simulink model "stage_2"  (Simulink 8.7)
settings: Solver=VariableStepAuto  StartTime=0.0  StopTime=inf  FixedStep=.000295  MaxStep=.0000118  RelTol=1e-3
settings Model: Creator=eispin  LastModifiedBy=eispin  PauseTimes=0
settings DataIOCC: LimitDataPoints=off  SaveFormat=Dataset
settings DebuggingCC: UnderspecifiedInitializationDetection=Simplified  MergeDetectMultiDrivingBlocksExec=error
settings HardwareCC: ProdBitPerPointer=64  ProdLargestAtomicFloat=Float  ProdIntDivRoundTo=Zero  ProdEndianess=LittleEndian  ProdWordSize=64  ProdHWDeviceType=Intel->x86-64 (Windows64)
settings ModelReferenceCC: PropagateSignalLabelsOutOfModel=on
settings ConfigComp: CovModelRefEnable=off

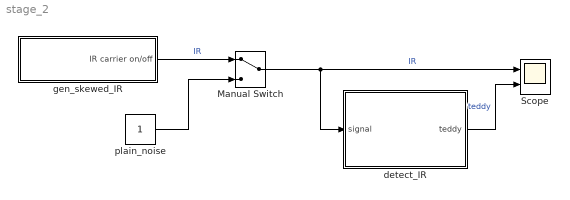
== system stage_2 ==
  Manual Switch : ManualSwitch
  Scope : Scope  NumInputPorts=2
  detect_IR : Stateflow chart  TreatAsAtomicUnit=on
  gen_skewed_IR : Subsystem
  plain_noise : Constant
  wires:
  Manual Switch/1 -> detect_IR/1(signal), Scope/1  "IR"
  detect_IR/1(teddy) -> Scope/2  "teddy"
  gen_skewed_IR/1(IR carrier on/off) -> Manual Switch/1  "IR"
  plain_noise/1 -> Manual Switch/2

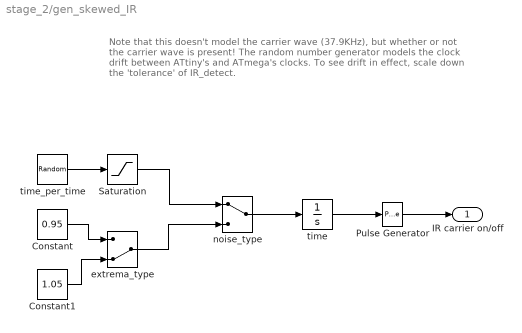
== system stage_2/gen_skewed_IR ==
  note: Note that this doesn't model the carrier wave (37.9KHz),
      | but whether or not the carrier wave is present!
      | The random number generator models the clock drift
      | between ATtiny's and ATmega's clocks.
      | To see drift in effect, scale down the 'tolerance' of IR_detect.
  Constant : Constant  Value=0.95
  Constant1 : Constant  Value=1.05
  Pulse Generator : DiscretePulseGenerator  PulseType=Time based  TimeSource=Use external signal  Period=.001180  PulseWidth=50
  Saturation : Saturate  UpperLimit=1.05  LowerLimit=0.95
  extrema_type : ManualSwitch  CurrentSetting=0
  noise_type : ManualSwitch
  time : Integrator
  time_per_time : RandomNumber  Mean=1  Variance=0.05  Seed=1337  SampleTime=0.000059
  IR carrier on/off : Outport
  wires:
  Pulse Generator/1 -> IR carrier on/off/1
  time/1 -> Pulse Generator/1
  time_per_time/1 -> Saturation/1
  noise_type/1 -> time/1
  Saturation/1 -> noise_type/1
  Constant/1 -> extrema_type/1
  extrema_type/1 -> noise_type/2
  Constant1/1 -> extrema_type/2

== stateflow chart detect_IR ==
  state NoTeddy
    % signal is 1,
    % waiting for 0
    entry:
    teddy = 0
  state Something
    % signal is 0,
    % waiting for 1
    entry:
    % don't change teddy
  note: Note that the "signal" must be treated as inverted,
      | so '0' is "carrier detected" and '1' is "carrier absent"
      | Tolerance:
      | - assume clock skew <= .1% (quartz has << .001%)
      |   => requirement:  tolerance >= .1% * 2 * pulse_length = 1.18µs
      | - assume that up to two periods of carrier are not detected in HW
      |   => requirement:  tolerance >= 2 * carrier_period = 53µs
      | Therefore, choose a tolerance of 60µs
      | => Accidentally allow clock skew up to 5%
  state WasTeddy
    % signal is 1
    % waiting for 0
    entry:
    teddy = 1
  state TooMuch
    % signal is 0,
    % waiting for 1
    entry:
    teddy = 0
  state ConfirmZero
  state ConfirmOne
  (default) -> NoTeddy
  ConfirmZero -> Something [order 1] : [after(590-tolerance, usec)]
  NoTeddy -> ConfirmZero : [signal < .5]
  ConfirmZero -> NoTeddy [order 2] : [signal > .5]
  WasTeddy -> ConfirmZero [order 2] : [signal < .5]
  Something -> ConfirmOne [order 2] : [signal > .5]
  Something -> TooMuch [order 1] : [after(2*tolerance, usec)]
  TooMuch -> NoTeddy : [signal > .5]
  WasTeddy -> NoTeddy [order 1] : [after(2*tolerance, usec)]
  ConfirmOne -> TooMuch [order 2] : [signal < .5]
  ConfirmOne -> WasTeddy [order 1] : [after(590-tolerance, usec)]
  data: signal input double; tolerance constant double =60; teddy output double
  data tolerance settings: description=MUST be bigger than the simulation stepsize
